simulink model "QuarterCar_AFC_v2"  (R2026a)
settings: Solver=ode4  StopTime=20  FixedStep=0.001
settings Model: Creator=Galaba Vamsi  LastModifiedBy=Galaba Vamsi

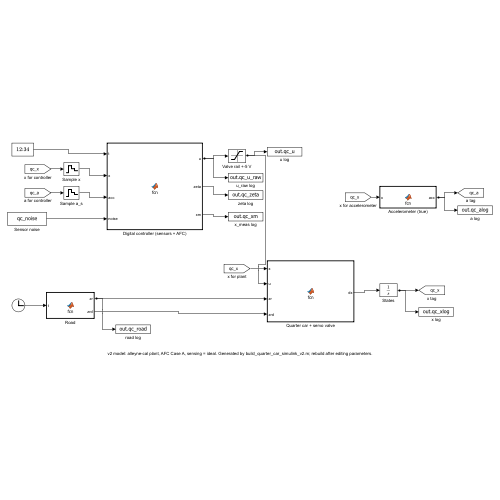
[thumbnail: Simulink's stored preview of the top-level diagram]
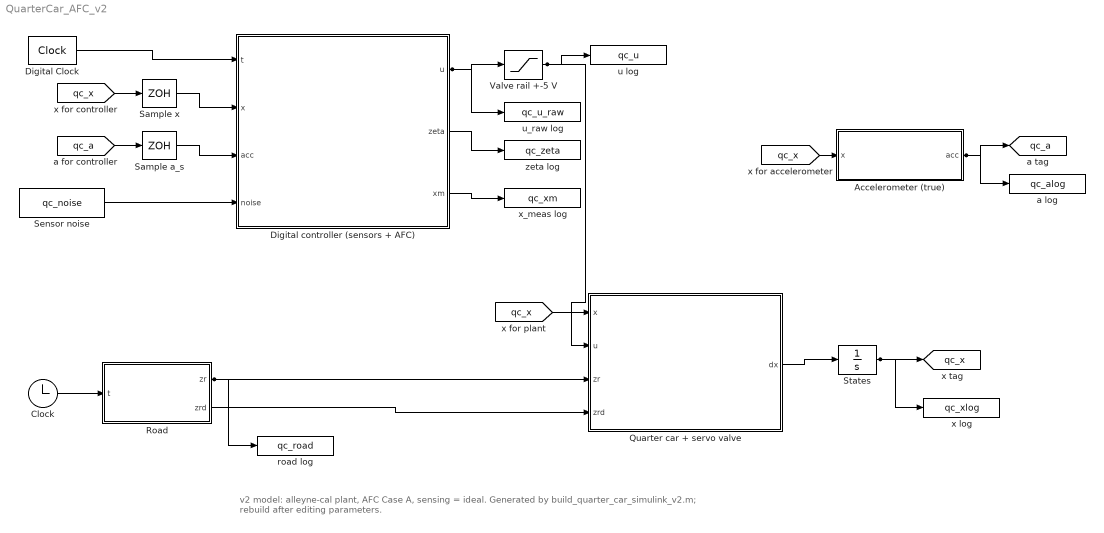
== system QuarterCar_AFC_v2 ==
  note: v2 model: alleyne-cal plant, AFC Case A, sensing = ideal. Generated by build_quarter_car_simulink_v2.m; rebuild after editing parameters.
  Accelerometer (true) : MATLAB Function  TreatAsAtomicUnit=on
  Clock : Clock
  Digital Clock : DigitalClock  SampleTime=0.02
  Digital controller (sensors + AFC) : MATLAB Function  TreatAsAtomicUnit=on
  Quarter car + servo valve : MATLAB Function  TreatAsAtomicUnit=on
  Road : MATLAB Function  TreatAsAtomicUnit=on
  Sample a_s : ZeroOrderHold  SampleTime=0.02
  Sample x : ZeroOrderHold  SampleTime=0.02
  Sensor noise : FromWorkspace  VariableName=qc_noise  SampleTime=0.02  Interpolate=off  OutputAfterFinalValue=Holding final value
  States : Integrator  InitialCondition=zeros(6,1)
  Valve rail +-5 V : Saturate  UpperLimit=5  LowerLimit=-5
  a log : ToWorkspace  VariableName=qc_alog  SaveFormat=Timeseries  SampleTime=-1
  road log : ToWorkspace  VariableName=qc_road  SaveFormat=Timeseries  SampleTime=-1
  u log : ToWorkspace  VariableName=qc_u  SaveFormat=Timeseries  SampleTime=-1
  u_raw log : ToWorkspace  VariableName=qc_u_raw  SaveFormat=Timeseries  SampleTime=-1
  x log : ToWorkspace  VariableName=qc_xlog  SaveFormat=Timeseries  SampleTime=-1
  x_meas log : ToWorkspace  VariableName=qc_xm  SaveFormat=Timeseries  SampleTime=-1
  zeta log : ToWorkspace  VariableName=qc_zeta  SaveFormat=Timeseries  SampleTime=-1
  tag scope: qc_a=global, qc_x=global
  wires:
  Clock/1 -> Road/1(t)
  Digital Clock/1 -> Digital controller (sensors + AFC)/1(t)
  [qc_x] -> Sample x/1
  Sample x/1 -> Digital controller (sensors + AFC)/2(x)
  [qc_a] -> Sample a_s/1
  Sample a_s/1 -> Digital controller (sensors + AFC)/3(acc)
  Sensor noise/1 -> Digital controller (sensors + AFC)/4(noise)
  Digital controller (sensors + AFC)/1(u) -> Valve rail +-5 V/1, u_raw log/1
  Digital controller (sensors + AFC)/2(zeta) -> zeta log/1
  Digital controller (sensors + AFC)/3(xm) -> x_meas log/1
  Valve rail +-5 V/1 -> u log/1, Quarter car + servo valve/2(u)
  [qc_x] -> Quarter car + servo valve/1(x)
  Road/1(zr) -> Quarter car + servo valve/3(zr), road log/1
  Road/2(zrd) -> Quarter car + servo valve/4(zrd)
  Quarter car + servo valve/1(dx) -> States/1
  States/1 -> [qc_x], x log/1
  [qc_x] -> Accelerometer (true)/1(x)
  Accelerometer (true)/1(acc) -> [qc_a], a log/1

== matlab function QuarterCar_AFC_v2/Digital controller (sensors + AFC) ==
  data: t input; u output; x input; acc input; noise input; zeta output; xm output
function [u, zeta, xm] = fcn(t, x, acc, noise)
% Runs at 50 Hz (sampled inputs). Sensors (mode 1: 1 ideal, 2 accint) + AFC eqs. (9)-(20)
persistent vInt
if isempty(vInt), vInt = 0; end
mode = 1; Ts = 0.02; lam = 0.9900498337491681;
sz = 0.0005; sa = 0.05; sp = 50000; kappa = 1e-06;
xm = x;
if mode == 2
  xm(1) = x(1) + sz*noise(1);
  vInt = lam*vInt + Ts*(acc + sa*noise(2));
  xm(2) = vInt;
  xm(5) = x(5) + kappa*sp*noise(3);
end
delta = 1; dbar = 1; g = 1e-08;
mu0 = [0.2; 110; 100]; muinf = [0.018; 90; 80];
al = [3; 2; 2]; k = [25.5; 12; 216];
mu = (mu0 - muinf).*exp(-al*t) + muinf;
src = [xm(1); xm(2); xm(5)];
zeta = zeros(3,1); prev = 0; v = 0;
for i = 1:3
  zeta(i) = (src(i) - prev)/mu(i);
  z = min(max(zeta(i), -delta + g), dbar - g);
  v = -k(i)*0.5*log((delta + z)/(dbar - z));
  prev = v;
end
u = v;
end

== matlab function QuarterCar_AFC_v2/Road ==
  data: t input; zr output; zrd output
function [zr, zrd] = fcn(t)
% Paper road case 10 peaks: 0.043 m, 0.505 Hz
A = 0.043; w = 3.173008580125691;
zr = A*sin(w*t);
zrd = A*w*cos(w*t);
end

== matlab function QuarterCar_AFC_v2/Quarter car + servo valve ==
  data: x input; u input; dx output; zr input; zrd input
function dx = fcn(x, u, zr, zrd)
% Quarter car (Na et al. eq. 7) + servo-valve flow law (eqs. 2-6) + spool lag
ms=290; mu=59; ks=16812; ksn=0; bs=1000; kt=190000; bt=0;
A=0.000335; alpha=45150000000000; beta=1; gamma=1545000000; Ps=10342500; kappa=1e-06; Kv=0.0005; tau=0.03333333333333333;
d=x(1)-x(3); v=x(2)-x(4);
Fs=ks*d+ksn*d^3; Fd=bs*v; Ft=kt*(x(3)-zr); Fb=bt*(x(4)-zrd);
PL=x(5)/kappa; F=A*PL;
dx=zeros(6,1);
if tau>0
  xv=x(6); dx(6)=(Kv*u-x(6))/tau;
else
  xv=Kv*u;
end
dP=Ps-sign(xv)*PL;
dx(5)=kappa*(-beta*PL-alpha*A*v+gamma*xv*sqrt(max(dP,0)));
dx(1)=x(2); dx(2)=(-Fd-Fs+F)/ms; dx(3)=x(4); dx(4)=(Fd+Fs-Ft-Fb-F)/mu;
end

== matlab function QuarterCar_AFC_v2/Accelerometer (true) ==
  data: x input; acc output
function acc = fcn(x)
% True body acceleration; depends on states only (no algebraic loop)
d=x(1)-x(3); v=x(2)-x(4);
acc=(-1000*v-(16812*d+0*d^3)+0.000335*x(5)/1e-06)/290;
end
